simulink model "improvedstopwatch"  (R2021a)
settings: Solver=VariableStepAuto  StartTime=0.0  StopTime=50  RelTol=1e-3
settings Model: EnablePacing=on  PacingRate=0.500000  Creator=kasra  LastModifiedBy=kasra

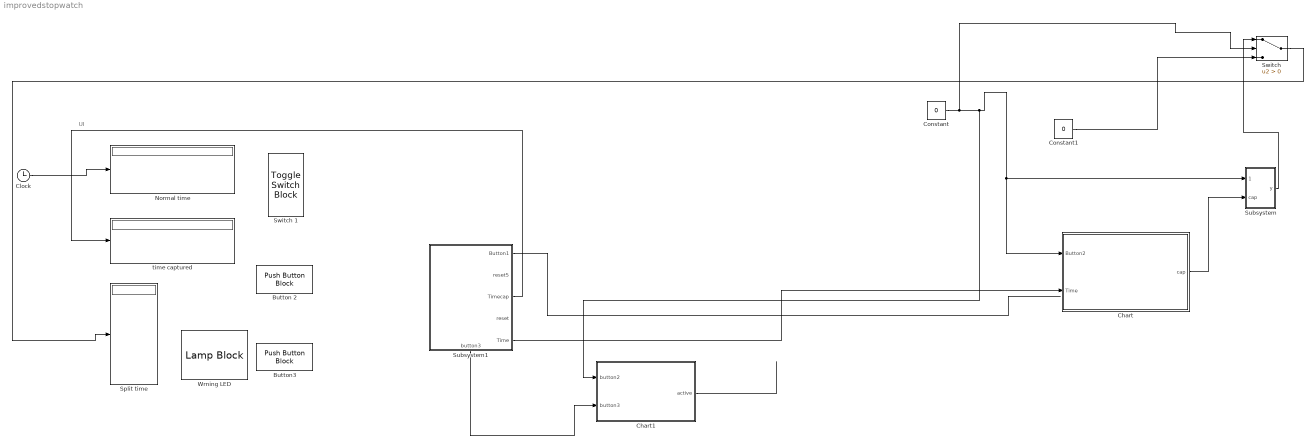
== system improvedstopwatch ==
  note: UI
  Button 2 : PushButtonBlock  ButtonText=Button2
  Button3 : PushButtonBlock  ButtonText=Reset
  Chart : Stateflow chart  TreatAsAtomicUnit=on
  Chart1 : Stateflow chart  TreatAsAtomicUnit=on
  Clock : Clock
      settings: Decimation=2
  Constant : Constant  Value=0
  Constant1 : Constant  Value=0
  Normal time : Display
  Split time : Display
  Subsystem : Subsystem
  Subsystem1 : Subsystem
      settings: PortSchema="{\"entries\":[{\"content\":{\"sides\":[{\"content\":{\"connectorIds\":[]},\"type\":\"ConnectorPlacement.EquallySpacedRectSide\",\"uuid\":\"21e32335-904f-44b9-a1bd-7c32fec6b7e4\"},{\"content\":{\"connectorIds\":[\"Out1\",\"Out2\",\"Out3\",\"Out4\",\"Out5\"],\"side\":\"RIGHT\"},\"type\":\"ConnectorPlacement.EquallySpacedRectSide\",\"uuid\":\"4bc76ca5-d21a-4374-a6fe-61bf81c89fd5\"},{\"content\":{\"connectorIds\":[],\"side\":\"TOP\"},\"type\":\"ConnectorPlacement.EquallySpacedRectSide\",\"uuid\":\"8460470b-f3bb-4249-b8f3-78a7eb61f6de\"},{\"content\":{\"connectorIds\":[\"Out6\"],\"side\":\"BOTTOM\"},\"type\":\"ConnectorPlacement.EquallySpacedRectSide\",\"uuid\":\"56fd258f-8091-44d5-86ab-ca4bff0ee104\"}]},\"type\":\"ConnectorPlacement.EquallySpacedConnector\",\"uuid\":\"bd0b3531-51ff-40ad-8be7-6b56c0bbb21d\"}],\"packageUris\":[\"http://schema.mathworks.com/mf0/Connector/R2020b\"],\"version\":\"1.0\"}"
  Switch : Switch  Criteria=u2 > Threshold
  Switch 1 : ToggleSwitchBlock
      settings: Values={{'Stop', 'Start'}, [1 0]}
  Wrning LED : LampBlock
  "time captured " : Display
  wires:
  Chart1/1(active) -> ?
  Chart/1(cap) -> Subsystem/2(cap)
  Constant/1 -> Switch/2, Chart1/1(button2), Subsystem/1(Trigger), Chart/1(Button2)
  Subsystem/1(y) -> Switch/1
  Subsystem1/5(Time) -> Chart/2(Time)
  Subsystem1/1(Button1) -> ?
  Subsystem1/6(button3) -> Chart1/2(button3)
  Switch/1 -> Split time/1
  Clock/1 -> Normal time/1
  Subsystem1/3(Timecap) -> "time captured "/1
  Constant1/1 -> Switch/3

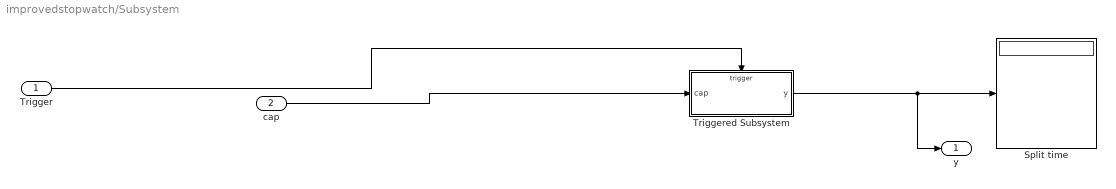
== system improvedstopwatch/Subsystem ==
  Trigger : Inport
  cap : Inport  Port=2
  Split time : Display
      settings: AttributesFormatString=%<RuntimeObject>
  Triggered Subsystem : Subsystem  TreatAsAtomicUnit=on
  y : Outport
  wires:
  Trigger/1 -> Triggered Subsystem/Trigger
  cap/1 -> Triggered Subsystem/1(cap)
  Triggered Subsystem/1(y) -> Split time/1, y/1

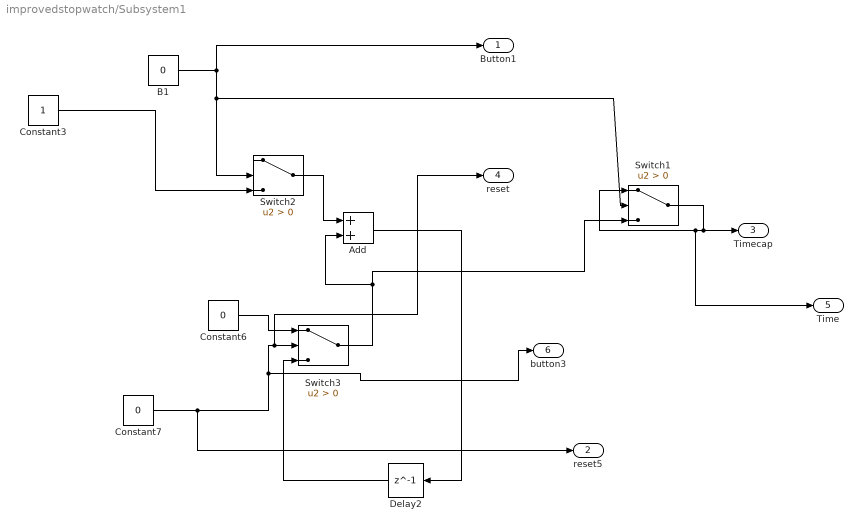
== system improvedstopwatch/Subsystem1 ==
  Add : Sum
  B1 : Constant  Value=0  VectorParams1D=off
  Constant3 : Constant
  Constant6 : Constant  Value=0
  Constant7 : Constant  Value=0
  Delay2 : Delay  DelayLength=1  InitialCondition=0  SampleTime=1
  Switch1 : Switch  Criteria=u2 > Threshold
  Switch2 : Switch  Criteria=u2 > Threshold
  Switch3 : Switch  Criteria=u2 > Threshold
  Button1 : Outport
  reset5 : Outport  Port=2
  Timecap : Outport  Port=3
  reset : Outport  Port=4
  Time : Outport  Port=5
  button3 : Outport  Port=6
  wires:
  Constant6/1 -> Switch3/1
  Switch3/1 -> Switch1/3, Add/2
  Add/1 -> Delay2/1
  Constant7/1 -> reset5/1, button3/1, reset/1, Switch3/2
  Delay2/1 -> Switch3/3
  B1/1 -> Switch2/2, Switch1/2, Button1/1
  Switch1/1 -> Time/1, Switch1/1, Timecap/1
  Constant3/1 -> Switch2/3
  Switch2/1 -> Add/1

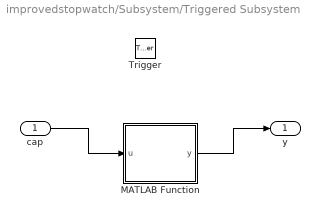
== system improvedstopwatch/Subsystem/Triggered Subsystem ==
  cap : Inport
  Trigger : TriggerPort  VariantControl=(inherit)
  MATLAB Function : MATLAB Function  TreatAsAtomicUnit=on
  y : Outport
  wires:
  cap/1 -> MATLAB Function/1(u)
  MATLAB Function/1(y) -> y/1

== stateflow chart improvedstopwatch/Chart1 ==
  state a
    entry:
    active = 0;
  state a1
    entry:
    active = 0
  state a2
    entry:
    active = 0
  state a3
    entry:
    active = 0
  state a4
    entry :
    active = 1;
  state a5
    entry:
    active = 0
  (default) -> a
  a1 -> a2 [order 1] : [button2 == 1]
  a2 -> (junction 15) [order 2] : [button3==1]
  a -> a1 : [button2 == 1]
  a5 -> a3 [order 1] : [button2 == 1]
  a3 -> a4 [order 1] : [button2 == 1]
  (junction 15) -> a
  a1 -> (junction 15) [order 2] : [button3==1]
  a3 -> (junction 15) [order 2] : [button3==1]
  a4 -> (junction 15) : [button3==1]
  a2 -> a5 [order 1] : [button2 == 1]
  a5 -> (junction 15) [order 2] : [button3==1]
  data: button2 input; active output; button3 input

== matlab function improvedstopwatch/Subsystem/Triggered Subsystem/MATLAB Function ==
  data: u input; y output
function y  = memory(u)
persistent slot
if isempty(slot) 
    slot = zeros(5,1);    
end
slot(2:end) = slot(1:end-1);
slot(1) = u(1);
y = slot;
if ~isempty(slot) 
    slot(5) = u(1)
end

== stateflow chart improvedstopwatch/Chart ==
  state Counter
    entry:
    Time
  state Capture1
    entry:
    cap = Time;
  (default) -> Counter
  Capture1 -> Counter : [Button2 == 0]
  Counter -> Capture1 : [Button2 == 1]
  data: Button2 input; Time input; cap output
